simulink model "sampleModel130"  (R2021b)
settings: Solver=VariableStepAuto  StartTime=0.0  StopTime=10.0  RelTol=1e-3
undefined symbols (not defined in the file or in its folder): Newton, Raphson
libraries: simulink x20, slpidlib x1
settings Model: Creator=user  LastModifiedBy=user

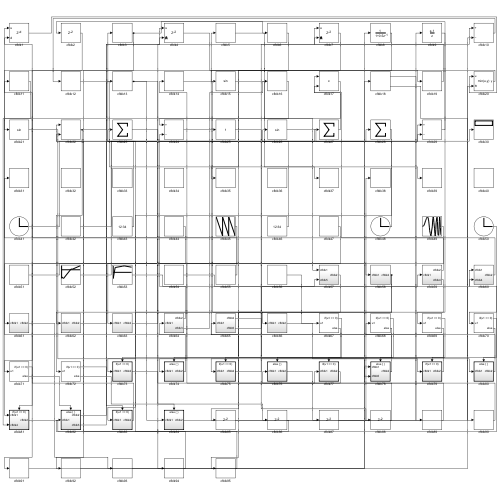
[thumbnail: Simulink's stored preview of the top-level diagram]
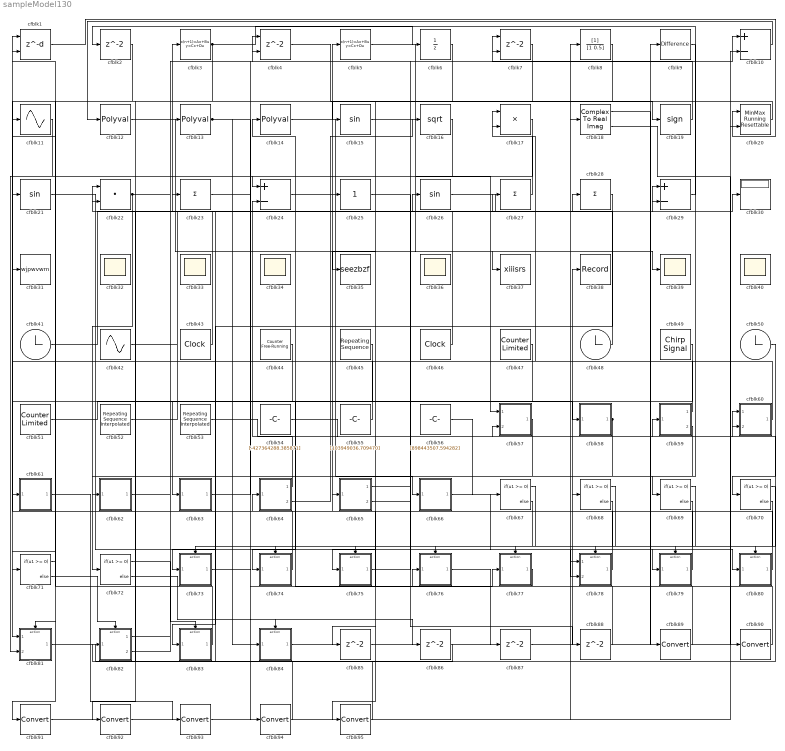
== system sampleModel130 ==
  cfblk1 : Delay  DelayLengthSource=Input port  SampleTime=1
      settings: InputPortMap=u0,p1
  cfblk10 : Sum  Inputs=+-
  cfblk11 : Sin  TimeSource=Use external signal  SampleTime=0
  cfblk12 : Polyval  Coefs=[ +2.081618890e-019, -1.441693666e-014, +4.719686976e-010, -8.536869453e-006, +1.621573104e-001, -8.087801117e+001 ]
  cfblk13 : Polyval  Coefs=[ +2.081618890e-019, -1.441693666e-014, +4.719686976e-010, -8.536869453e-006, +1.621573104e-001, -8.087801117e+001 ]
  cfblk14 : Polyval  Coefs=[ +2.081618890e-019, -1.441693666e-014, +4.719686976e-010, -8.536869453e-006, +1.621573104e-001, -8.087801117e+001 ]
  cfblk15 : Trigonometry
  cfblk16 : Sqrt  SaturateOnIntegerOverflow=on
  cfblk17 : Product
  cfblk18 : ComplexToRealImag
  cfblk19 : Signum
  cfblk{2,85..88} (5 alike) : Delay  SampleTime=1
  cfblk20 : simulink/Math Operations/MinMax Running Resettable  Function=min  vinit=0.0
  cfblk21 : Trigonometry
  cfblk22 : DotProduct  InputSameDT=on  OutDataTypeStr=Inherit: Inherit via internal rule
  cfblk23 : Sum  Inputs=+
  cfblk24 : Sum  Inputs=+-
  cfblk25 : simulink/Math Operations/Slider Gain  gain=1  low=0  high=2
  cfblk26 : Trigonometry
  cfblk27 : Sum  Inputs=+
  cfblk28 : Sum  Inputs=+
  cfblk29 : Sum  Inputs=+-
  cfblk3 : DiscreteStateSpace
  cfblk30 : Display
  cfblk31 : ToWorkspace  VariableName=wjpwvwm  SaveFormat=Timeseries  SampleTime=-1
  cfblk{32..34,36,39..40} (6 alike) : Scope
      cfblk32 settings: Floating=on
      cfblk33 settings: Floating=on
      cfblk34 settings: Floating=on
      cfblk36 settings: Floating=on
      cfblk40 settings: Floating=on
  cfblk35 : ToWorkspace  VariableName=seezbzf  SaveFormat=Timeseries  SampleTime=-1
  cfblk37 : ToWorkspace  VariableName=xiiisrs  SaveFormat=Timeseries  SampleTime=-1
  cfblk38 : Record  FileSettingsInternal="{\"entries\":[{\"content\":{\"excelSettings\":{\"content\":{},\"type\":\"Streamout.ExcelSettings\"}},\"type\":\"Streamout.FileSettingStorage\",\"uuid\":\"df2d4dfc-2a52-453f-9162-7e4b7b1ef560\"}],\"packageUris\":[\"http://schema.mathworks.com/mf0/streamout_blocks/R2020a\"],\"version\":\"1.0\"}"  SignalsInternal="{\"entries\":[{\"content\":{\"signals\":[{\"content\":{\"blockPath\":[\"sampleModel130/cfblk38\"],\"channel\":[],\"dimensions\":[1],\"domain\":\"sampleModel130/cfblk38\",\"lineColor\":\"#ff6929\",\"plots\":[1],\"port\":1,\"sid\":[\"\"],\"signalID\":4547,\"signalName\":\"cfblk84\"},\"type\":\"RecordBlkView.Signal\",\"uuid\":\"77a7a94c-391c-43bd-ba92-53a2dba3dce4\"}]},\"type\":\"RecordBlkView.InputSignals\",\"uuid\":\"1134eac6-1b87-41a8-a267-5a408cb23513\"}],\"packageUris\":[\"http://schema.mathworks.com/mf0/streamout_blocks/R2020a\"],\"version\":\"1.0\"}"  VisualizationBindings="{\"sparklinesplugin\":{\"info\":[{\"bindingParametersList\":[],\"subplotID\":1}]}}"
  cfblk4 : Delay  ShowEnablePort=on  SampleTime=1
      settings: InputPortMap=u0,e6
  cfblk41 : Clock
  cfblk42 : Sin  Amplitude=[-790719312.220439]  Bias=[400958041.648387]  SampleTime=0
  cfblk43 : DigitalClock
  cfblk44 : simulink/Sources/Counter Free-Running  NumBits=[5.000000]  tsamp=-1
  cfblk45 : simulink/Sources/Repeating Sequence  rep_seq_t=[0 2]  rep_seq_y=[782391046.250394, 387760323.492040]
  cfblk46 : DigitalClock
  cfblk47 : simulink/Sources/Counter Limited  uplimit=[437.000000]  tsamp=-1
  cfblk48 : Clock
  cfblk49 : simulink/Sources/Chirp Signal  f1=[313982218.934248]  T=[896188493.416858]  f2=[542107729.166692]
  cfblk5 : DiscreteStateSpace
  cfblk50 : Clock
  cfblk51 : simulink/Sources/Counter Limited  uplimit=[883.000000]  tsamp=-1
  cfblk52 : simulink/Sources/Repeating Sequence Interpolated  OutValues=[-314051467.963771, -374670403.765371, 15377636.426483, 25046100.552670, 163693646.781448]  TimeValues=[0 0.1 0.5 0.6 1].'  LookUpMeth=Use Input Nearest  tsamp=0.01  OutMin=[]  OutMax=[]  OutDataTypeStr=double  OutputDataTypeScalingMode=double  OutDataType=fixdt(0,8)  OutScaling=2^-10
  cfblk53 : simulink/Sources/Repeating Sequence Interpolated  OutValues=[-518560608.877954, 432871116.350142, 539806511.247294, 582480267.975265, 460023468.069956]  TimeValues=[0 0.1 0.5 0.6 1].'  LookUpMeth=Interpolation-Use End Values  tsamp=0.01  OutMin=[]  OutMax=[]  OutDataTypeStr=double  OutputDataTypeScalingMode=double  OutDataType=fixdt(0,8)  OutScaling=2^-10
  cfblk54 : Constant  Value=[-427364288.385871]  SampleTime=1
  cfblk55 : Constant  Value=[103949036.709470]  SampleTime=1
  cfblk56 : Constant  Value=[898443507.594282]  SampleTime=1
  cfblk57 : Subsystem
  cfblk58 : Subsystem
  cfblk59 : Subsystem
  cfblk6 : UnitDelay  HasFrameUpgradeWarning=on
  cfblk60 : Subsystem
  cfblk61 : Subsystem
  cfblk62 : Subsystem
  cfblk63 : Subsystem
  cfblk64 : Subsystem
  cfblk65 : Subsystem
  cfblk66 : Subsystem
  cfblk{67..72} (6 alike) : If  IfExpression=u1 >= 0  SampleTime=1
  cfblk7 : Delay  ShowEnablePort=on  SampleTime=1
      settings: InputPortMap=u0,e6
  cfblk73 : Subsystem  TreatAsAtomicUnit=on
  cfblk74 : Subsystem  TreatAsAtomicUnit=on
  cfblk75 : Subsystem  TreatAsAtomicUnit=on
  cfblk76 : Subsystem  TreatAsAtomicUnit=on
  cfblk77 : Subsystem  TreatAsAtomicUnit=on
  cfblk78 : Subsystem  TreatAsAtomicUnit=on
  cfblk79 : Subsystem  TreatAsAtomicUnit=on
  cfblk8 : DiscreteFilter  SampleTime=1
  cfblk80 : Subsystem  TreatAsAtomicUnit=on
  cfblk81 : Subsystem  TreatAsAtomicUnit=on
  cfblk82 : Subsystem  TreatAsAtomicUnit=on
  cfblk83 : Subsystem  TreatAsAtomicUnit=on
  cfblk84 : Subsystem  TreatAsAtomicUnit=on
  cfblk{89..95} (7 alike) : DataTypeConversion
  cfblk9 : simulink/Discrete/Difference  ICPrevInput=0.0  OutMin=[]  OutMax=[]  OutDataTypeStr=Inherit: Inherit via back propagation  OutDataType=fixdt(1, 16)  OutScaling=2^-10  DoSatur=off
  wires:
  cfblk79/1(cfblk2) -> cfblk5/1
  cfblk56/1 -> cfblk67/1
  cfblk84/1(cfblk2) -> cfblk38/1
  cfblk29/1 -> cfblk2/1
  cfblk55/1 -> cfblk1/1
  cfblk45/1 -> cfblk63/1(cfblk1)
  cfblk14/1 -> cfblk66/1(cfblk1)
  cfblk10/1 -> cfblk12/1
  cfblk5/1 -> cfblk39/1
  cfblk11/1 -> cfblk81/1(cfblk1)
  cfblk74/1(cfblk2) -> cfblk31/1
  cfblk2/1 -> cfblk21/1
  cfblk27/1 -> cfblk17/1
  cfblk66/1(cfblk2) -> cfblk80/1(cfblk1)
  cfblk9/1 -> cfblk69/1
  cfblk26/1 -> cfblk28/1
  cfblk81/1(cfblk2) -> cfblk60/1(cfblk1)
  cfblk51/1 -> cfblk58/1(cfblk1)
  cfblk12/1 -> cfblk37/1
  cfblk47/1 -> cfblk61/1(cfblk1)
  cfblk3/1 -> cfblk6/1, cfblk71/1
  cfblk48/1 -> cfblk26/1
  cfblk60/1(cfblk2) -> cfblk1/2
  cfblk83/1(cfblk2) -> cfblk11/1
  cfblk28/1 -> cfblk83/1(cfblk1)
  cfblk16/1 -> cfblk81/2(cfblk4)
  cfblk19/1 -> cfblk7/1
  cfblk4/1 -> cfblk19/1
  cfblk80/1(cfblk2) -> cfblk64/1(cfblk1)
  cfblk43/1 -> cfblk3/1
  cfblk65/1(cfblk2) -> cfblk78/2(cfblk5)
  cfblk49/1 -> cfblk74/1(cfblk1)
  cfblk59/1(cfblk2) -> cfblk17/2
  cfblk20/1 -> cfblk15/1
  cfblk82/1(cfblk2) -> cfblk13/1
  cfblk58/1(cfblk2) -> cfblk75/1(cfblk1), cfblk73/1(cfblk1)
  cfblk54/1 -> cfblk60/2(cfblk4)
  cfblk52/1 -> cfblk29/1
  cfblk17/1 -> cfblk24/1
  cfblk77/1(cfblk2) -> cfblk76/1(cfblk1)
  cfblk24/1 -> cfblk25/1
  cfblk15/1 -> cfblk57/1(cfblk1)
  cfblk13/1 -> cfblk84/1(cfblk1), cfblk86/1
  cfblk75/1(cfblk2) -> cfblk59/1(cfblk1)
  cfblk41/1 -> cfblk27/1
  cfblk46/1 -> cfblk22/1
  cfblk22/1 -> cfblk72/1, cfblk4/2
  cfblk21/1 -> cfblk79/1(cfblk1)
  cfblk6/1 -> cfblk35/1
  cfblk82/2(cfblk3) -> cfblk29/2
  cfblk65/2(cfblk5) -> cfblk10/1
  cfblk53/1 -> cfblk57/2(cfblk5)
  cfblk64/1(cfblk2) -> cfblk24/2
  cfblk63/1(cfblk2) -> cfblk7/2
  cfblk62/1(cfblk2) -> cfblk4/1
  cfblk57/1(cfblk2) -> cfblk62/1(cfblk1)
  cfblk50/1 -> cfblk70/1
  cfblk42/1 -> cfblk30/1
  cfblk64/2(cfblk3) -> cfblk16/1
  cfblk78/1(cfblk2) -> cfblk68/1
  cfblk1/1 -> cfblk20/1
  cfblk73/1(cfblk2) -> cfblk77/1(cfblk1)
  cfblk67/1 -> cfblk73/Action
  cfblk67/2 -> cfblk74/Action
  cfblk68/1 -> cfblk75/Action
  cfblk68/2 -> cfblk76/Action
  cfblk69/1 -> cfblk77/Action
  cfblk69/2 -> cfblk78/Action
  cfblk70/1 -> cfblk79/Action
  cfblk70/2 -> cfblk80/Action
  cfblk71/1 -> cfblk81/Action
  cfblk71/2 -> cfblk82/Action
  cfblk72/1 -> cfblk83/Action
  cfblk72/2 -> cfblk84/Action
  cfblk7/1 -> cfblk85/1
  cfblk85/1 -> cfblk20/2
  cfblk86/1 -> cfblk82/1(cfblk1)
  cfblk76/1(cfblk2) -> cfblk87/1
  cfblk87/1 -> cfblk9/1
  cfblk25/1 -> cfblk88/1
  cfblk88/1 -> cfblk78/1(cfblk1)
  cfblk18/1 -> cfblk89/1
  cfblk89/1 -> cfblk65/1(cfblk1)
  cfblk18/2 -> cfblk90/1
  cfblk90/1 -> cfblk14/1
  cfblk44/1 -> cfblk91/1
  cfblk91/1 -> cfblk18/1
  cfblk8/1 -> cfblk92/1
  cfblk92/1 -> cfblk10/2
  cfblk61/1(cfblk2) -> cfblk93/1
  cfblk93/1 -> cfblk8/1
  cfblk23/1 -> cfblk94/1
  cfblk94/1 -> cfblk22/2
  cfblk59/2(cfblk4) -> cfblk95/1
  cfblk95/1 -> cfblk23/1

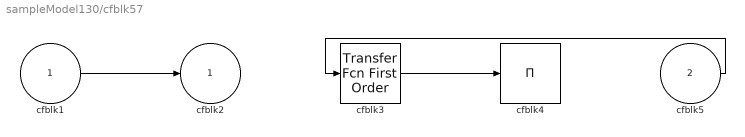
== system sampleModel130/cfblk57 ==
  cfblk1 : Inport
  cfblk5 : Inport  Port=2
  cfblk3 : simulink/Discrete/Transfer Fcn First Order  PoleZ=0.95  ICPrevOutput=0.0  DoSatur=off
  cfblk4 : Product  Inputs=*
  cfblk2 : Outport
  wires:
  cfblk3/1 -> cfblk4/1
  cfblk5/1 -> cfblk3/1
  cfblk1/1 -> cfblk2/1

== system sampleModel130/cfblk58 ==
  cfblk1 : Inport
  cfblk3 : Product  Inputs=*
  cfblk2 : Outport
  wires:
  cfblk1/1 -> cfblk2/1, cfblk3/1

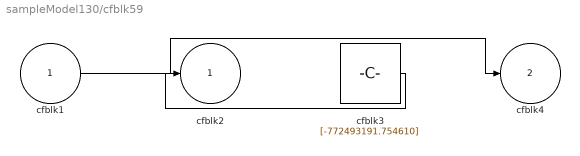
== system sampleModel130/cfblk59 ==
  cfblk1 : Inport
  cfblk3 : Constant  Value=[-772493191.754610]  SampleTime=1
  cfblk2 : Outport
  cfblk4 : Outport  Port=2
  wires:
  cfblk1/1 -> cfblk4/1
  cfblk3/1 -> cfblk2/1

== system sampleModel130/cfblk60 ==
  cfblk1 : Inport
  cfblk4 : Inport  Port=2
  cfblk3 : Product
  cfblk2 : Outport
  wires:
  cfblk1/1 -> cfblk3/1
  cfblk4/1 -> cfblk3/2
  cfblk3/1 -> cfblk2/1

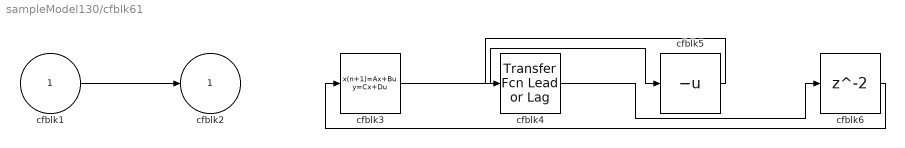
== system sampleModel130/cfblk61 ==
  cfblk1 : Inport
  cfblk3 : DiscreteStateSpace
  cfblk4 : simulink/Discrete/Transfer Fcn Lead or Lag  PoleZ=0.95  ZeroZ=0.75  ICPrevOutput=0.0  ICPrevInput=0.0  DoSatur=off
      settings: SourceProductBaseCode=SL
  cfblk5 : UnaryMinus
  cfblk6 : Delay  SampleTime=1
  cfblk2 : Outport
  wires:
  cfblk3/1 -> cfblk5/1
  cfblk1/1 -> cfblk2/1
  cfblk5/1 -> cfblk4/1
  cfblk4/1 -> cfblk6/1
  cfblk6/1 -> cfblk3/1

== system sampleModel130/cfblk62 ==
  cfblk1 : Inport
  cfblk3 : Constant  Value=[-333365384.204087]  SampleTime=1
  cfblk2 : Outport
  wires:
  cfblk3/1 -> cfblk2/1

== system sampleModel130/cfblk63 ==
  cfblk1 : Inport
  cfblk3 : simulink/Discrete/Transfer Fcn First Order  PoleZ=0.95  ICPrevOutput=0.0  DoSatur=off
  cfblk4 : Assignment  DiagnosticForDimensions=Warning  IndexOptions=Index vector (dialog)  Indices=1  OutputSizes=1
  cfblk2 : Outport
  wires:
  cfblk3/1 -> cfblk2/1
  cfblk4/1 -> cfblk3/1
  cfblk1/1 -> cfblk4/1, cfblk4/2

== system sampleModel130/cfblk64 ==
  cfblk1 : Inport
  cfblk2 : Outport
  cfblk3 : Outport  Port=2
  wires:
  cfblk1/1 -> cfblk2/1, cfblk3/1

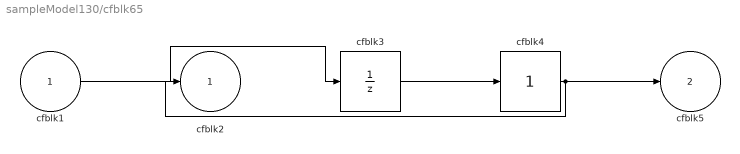
== system sampleModel130/cfblk65 ==
  cfblk1 : Inport
  cfblk3 : UnitDelay  HasFrameUpgradeWarning=on
  cfblk4 : simulink/Math Operations/Slider Gain  gain=1  low=0  high=2
  cfblk2 : Outport
  cfblk5 : Outport  Port=2
  wires:
  cfblk1/1 -> cfblk3/1
  cfblk4/1 -> cfblk2/1, cfblk5/1
  cfblk3/1 -> cfblk4/1

== system sampleModel130/cfblk66 ==
  cfblk1 : Inport
  cfblk3 : DiscreteFir  SampleTime=1
  cfblk2 : Outport
  wires:
  cfblk1/1 -> cfblk3/1
  cfblk3/1 -> cfblk2/1

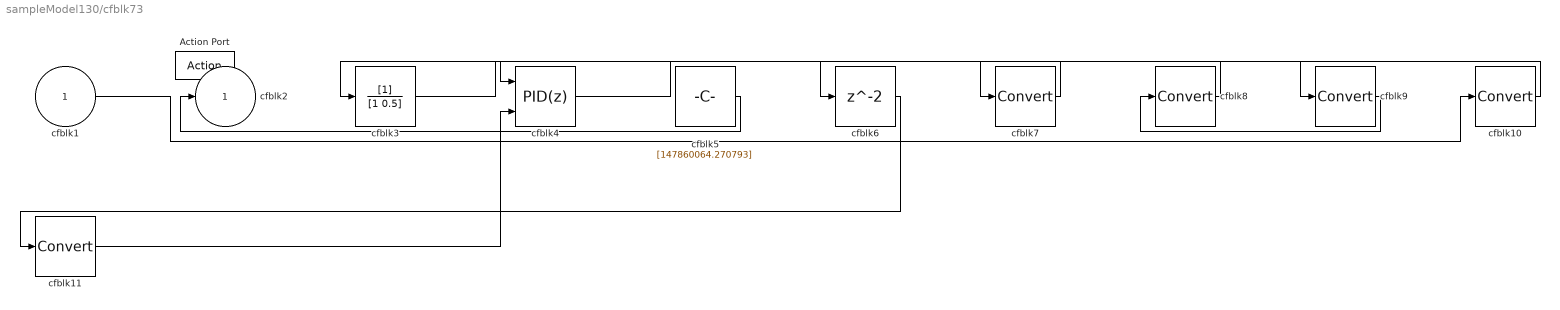
== system sampleModel130/cfblk73 ==
  cfblk1 : Inport
  Action Port : ActionPort  ActionPortLabel=if(u1 >= 0)
  cfblk{7..11} (5 alike) : DataTypeConversion
  cfblk3 : DiscreteFilter
  cfblk4 : slpidlib/PID Controller (2DOF)  Controller=PID  Form=Parallel  TimeDomain=Discrete-time  UseExternalTs=off  SampleTime=-1  IntegratorMethod=Forward Euler  FilterMethod=Forward Euler  ControllerParametersSource=internal  P=1  I=1  D=0  UseFilter=on  N=100  b=1  c=1  TunerSelectOption=Transfer Function Based (PID Tuner App)  InitialConditionSource=internal  InitialConditionForIntegrator=0  InitialConditionForFilter=0  DifferentiatorICPrevScaledInput=0  ExternalReset=none  TrackingMode=off  Kt=1  LimitOutput=off  SatLimitsSource=internal  UpperSaturationLimit=inf  LowerSaturationLimit=-inf  LinearizeAsGain=off  AntiWindupMode=none  Kb=1  POutMin=[]  POutMax=[]  IOutMin=[]  IOutMax=[]  DOutMin=[]  DOutMax=[]  NOutMin=[]  NOutMax=[]  bOutMin=[]  bOutMax=[]  cOutMin=[]  cOutMax=[]  SumOutMin=[]  SumOutMax=[]  SaturationOutMin=[]  SaturationOutMax=[]  PParamMin=[]  PParamMax=[]  IParamMin=[]  IParamMax=[]  DParamMin=[]  DParamMax=[]  NParamMin=[]  NParamMax=[]  bParamMin=[]  bParamMax=[]  cParamMin=[]  cParamMax=[]  KbParamMin=[]  KbParamMax=[]  KtParamMin=[]  KtParamMax=[]  KbOutMin=[]  KbOutMax=[]  KtOutMin=[]  KtOutMax=[]  IntegratorOutMin=[]  IntegratorOutMax=[]  FilterOutMin=[]  FilterOutMax=[]  SumI1OutMin=[]  SumI1OutMax=[]  SumI2OutMin=[]  SumI2OutMax=[]  SumI3OutMin=[]  SumI3OutMax=[]  SumI4OutMin=[]  SumI4OutMax=[]  SumDOutMin=[]  SumDOutMax=[]  Sum1OutMin=[]  Sum1OutMax=[]  Sum2OutMin=[]  Sum2OutMax=[]  Sum3OutMin=[]  Sum3OutMax=[]  DifferentiatorOutMin=[]  DifferentiatorOutMax=[]  FilterDiffOutCoefMin=[]  FilterDiffOutCoefMax=[]  ReciprocalOutMin=[]  ReciprocalOutMax=[]  SumDenOutMin=[]  SumDenOutMax=[]  SumNumOutMin=[]  SumNumOutMax=[]  DivideOutMin=[]  DivideOutMax=[]  UdiffTsProdOutMin=[]  UdiffTsProdOutMax=[]  NTsProdOutMin=[]  NTsProdOutMax=[]  UintegralTsProdOutMin=[]  UintegralTsProdOutMax=[]  UngainTsProdOutMin=[]  UngainTsProdOutMax=[]  IntegratorContinuousStateAttributes=''  IntegratorStateMustResolveToSignalObject=off  IntegratorRTWStateStorageClass=Auto  FilterContinuousStateAttributes=''  FilterStateMustResolveToSignalObject=off  FilterRTWStateStorageClass=Auto  ParallelPVariant=InternalParameters  IdealPVariant=Disabled  IVariant=InternalParameters  DVariant=InternalParameters  bVariant=InternalParameters  cVariant=InternalParameters  IntegratorVariant=Discrete  SatVariant=Disabled  AWVariant=Passthrough  PCopyVariant=Disabled  TRVariant=Disabled  FdbkBlocksVariant=Forward  IdealPFdbkVariant=Disabled  SatFdbkVariant=Disabled  DerivativeFilterVariant=ForwardEulerFilter  NVariant=InternalParameters  NCopyVariant=Disabled  FilterICVariant=InternalICsFilter  IntegratorICVariant=InternalICs  ExternalResetVariant=Disabled  TRSumVariant=Passthrough  SumFdbkVariant=Disabled  SumVariant=Sum_PID  TsampFilterVariant=InternalTs  TsampNgainVariant=Passthrough  TsampIntegralVariant=Passthrough  ExternalSaturationOutDataTypeStr=Inherit: Same as second input
      settings: SourceProductBaseCode=SL
  cfblk5 : Constant  Value=[147860064.270793]  SampleTime=1
  cfblk6 : Delay
  cfblk2 : Outport
  wires:
  cfblk5/1 -> cfblk2/1
  cfblk3/1 -> cfblk7/1
  cfblk7/1 -> cfblk6/1
  cfblk8/1 -> cfblk3/1
  cfblk4/1 -> cfblk9/1
  cfblk9/1 -> cfblk8/1
  cfblk1/1 -> cfblk10/1
  cfblk10/1 -> cfblk4/1
  cfblk6/1 -> cfblk11/1
  cfblk11/1 -> cfblk4/2

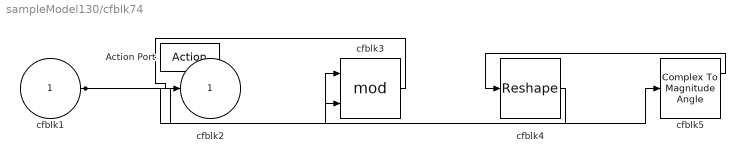
== system sampleModel130/cfblk74 ==
  cfblk1 : Inport
  Action Port : ActionPort  ActionPortLabel=else
  cfblk3 : Math  Operator=mod  SaturateOnIntegerOverflow=on
  cfblk4 : Reshape
  cfblk5 : ComplexToMagnitudeAngle
  cfblk2 : Outport
  wires:
  cfblk1/1 -> cfblk3/1, cfblk5/1
  cfblk4/1 -> cfblk3/2
  cfblk3/1 -> cfblk2/1
  cfblk5/1 -> cfblk4/1

== system sampleModel130/cfblk75 ==
  cfblk1 : Inport
  Action Port : ActionPort  ActionPortLabel=if(u1 >= 0)
  cfblk3 : simulink/Math Operations/Slider Gain  gain=1  low=0  high=2
  cfblk2 : Outport
  wires:
  cfblk3/1 -> cfblk2/1
  cfblk1/1 -> cfblk3/1

== system sampleModel130/cfblk76 ==
  cfblk1 : Inport
  Action Port : ActionPort  ActionPortLabel=else
  cfblk3 : Delay  ShowEnablePort=on
      settings: InputPortMap=u0,e6
  cfblk2 : Outport
  wires:
  cfblk3/1 -> cfblk2/1
  cfblk1/1 -> cfblk3/1, cfblk3/2

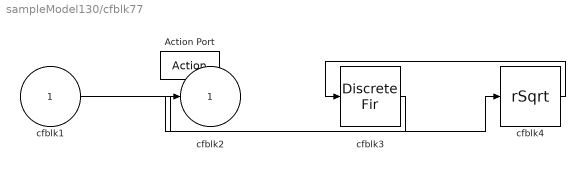
== system sampleModel130/cfblk77 ==
  cfblk1 : Inport
  Action Port : ActionPort  ActionPortLabel=if(u1 >= 0)
  cfblk3 : DiscreteFir
  cfblk4 : Sqrt  Operator=rSqrt  AlgorithmType=Newton-Raphson  SaturateOnIntegerOverflow=on
  cfblk2 : Outport
  wires:
  cfblk4/1 -> cfblk3/1
  cfblk1/1 -> cfblk4/1
  cfblk3/1 -> cfblk2/1

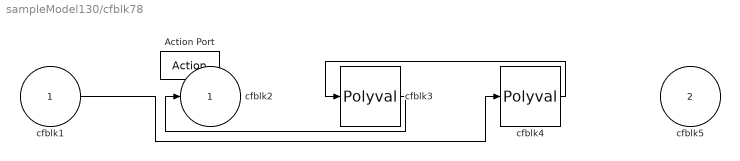
== system sampleModel130/cfblk78 ==
  cfblk1 : Inport
  cfblk5 : Inport  Port=2
  Action Port : ActionPort  ActionPortLabel=else
  cfblk3 : Polyval  Coefs=[ +2.081618890e-019, -1.441693666e-014, +4.719686976e-010, -8.536869453e-006, +1.621573104e-001, -8.087801117e+001 ]
  cfblk4 : Polyval  Coefs=[ +2.081618890e-019, -1.441693666e-014, +4.719686976e-010, -8.536869453e-006, +1.621573104e-001, -8.087801117e+001 ]
  cfblk2 : Outport
  wires:
  cfblk3/1 -> cfblk2/1
  cfblk4/1 -> cfblk3/1
  cfblk1/1 -> cfblk4/1

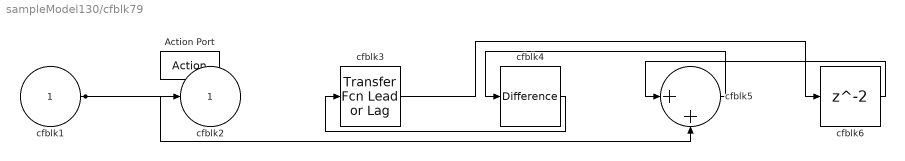
== system sampleModel130/cfblk79 ==
  cfblk1 : Inport
  Action Port : ActionPort  ActionPortLabel=if(u1 >= 0)
  cfblk3 : simulink/Discrete/Transfer Fcn Lead or Lag  PoleZ=0.95  ZeroZ=0.75  ICPrevOutput=0.0  ICPrevInput=0.0  DoSatur=off
      settings: SourceProductBaseCode=SL
  cfblk4 : simulink/Discrete/Difference  ICPrevInput=0.0  OutMin=[]  OutMax=[]  OutDataTypeStr=Inherit: Inherit via back propagation  OutDataType=fixdt(1, 16)  OutScaling=2^-10  DoSatur=off
  cfblk5 : Sum  Inputs=|++
  cfblk6 : Delay
  cfblk2 : Outport
  wires:
  cfblk4/1 -> cfblk3/1
  cfblk1/1 -> cfblk2/1, cfblk5/2
  cfblk5/1 -> cfblk4/1
  cfblk3/1 -> cfblk6/1
  cfblk6/1 -> cfblk5/1

== system sampleModel130/cfblk80 ==
  cfblk1 : Inport
  Action Port : ActionPort  ActionPortLabel=else
  cfblk3 : simulink/Math Operations/Slider Gain  gain=1  low=0  high=2
  cfblk2 : Outport
  wires:
  cfblk1/1 -> cfblk2/1, cfblk3/1

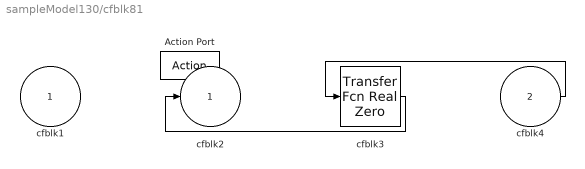
== system sampleModel130/cfblk81 ==
  cfblk1 : Inport
  cfblk4 : Inport  Port=2
  Action Port : ActionPort  ActionPortLabel=if(u1 >= 0)
  cfblk3 : simulink/Discrete/Transfer Fcn Real Zero  ZeroZ=0.75  ICPrevInput=0.0  DoSatur=off
      settings: SourceProductBaseCode=SL
  cfblk2 : Outport
  wires:
  cfblk3/1 -> cfblk2/1
  cfblk4/1 -> cfblk3/1

== system sampleModel130/cfblk82 ==
  cfblk1 : Inport
  Action Port : ActionPort  ActionPortLabel=else
  cfblk2 : Outport
  cfblk3 : Outport  Port=2
  wires:
  cfblk1/1 -> cfblk3/1, cfblk2/1

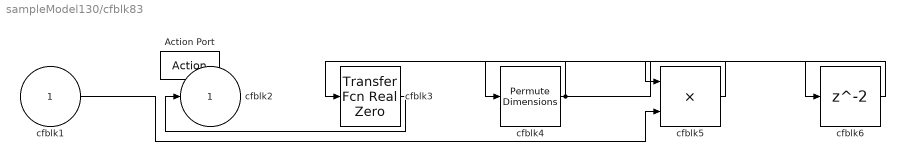
== system sampleModel130/cfblk83 ==
  cfblk1 : Inport
  Action Port : ActionPort  ActionPortLabel=if(u1 >= 0)
  cfblk3 : simulink/Discrete/Transfer Fcn Real Zero  ZeroZ=0.75  ICPrevInput=0.0  DoSatur=off
      settings: SourceProductBaseCode=SL
  cfblk4 : PermuteDimensions
  cfblk5 : Product
  cfblk6 : Delay
  cfblk2 : Outport
  wires:
  cfblk4/1 -> cfblk3/1, cfblk6/1
  cfblk3/1 -> cfblk2/1
  cfblk1/1 -> cfblk5/2
  cfblk5/1 -> cfblk4/1
  cfblk6/1 -> cfblk5/1

== system sampleModel130/cfblk84 ==
  cfblk1 : Inport
  Action Port : ActionPort  ActionPortLabel=else
  cfblk3 : Product  Inputs=**
  cfblk2 : Outport
  wires:
  cfblk1/1 -> cfblk2/1, cfblk3/1, cfblk3/2
